simulink model "simulink_jacoviano"  (R2018b)
settings: Solver=VariableStepAuto  StartTime=0.0  StopTime=10.0  RelTol=1e-3
settings Model: Creator=aland  LastModifiedBy=aland

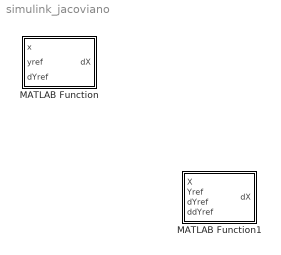
== system simulink_jacoviano ==
  MATLAB Function : MATLAB Function  TreatAsAtomicUnit=on
  MATLAB Function1 : MATLAB Function  TreatAsAtomicUnit=on

== matlab function simulink_jacoviano/MATLAB Function1 ==
  data: X input; dX output; Yref input; dYref input; ddYref input
function dX = simulink_motor(X, Yref, dYref, ddYref)

%MATRICES DEL MOTOR
Ra = 11.24;
La = 2.713e-3;
Kb = 14.87e-3;
Kt = Kb;
bm = 2.01e-6;
Jm = 2779.56e-9;

A = [-Ra/La -Kb/La;Kt/Jm -bm/Jm];
B = [1/La;0];
C = [0 1];

x1 = X(1); x2 = X(2);

e2 = Yref - x2;
de2 = dYref - (Kt/Jm)*x1 + (bm/Jm)*x2;

X1ref = (Jm/Kt)*(dYref + (bm/Jm)*x2 - k2*e2);
dX1ref = (Jm/Kt)*(-k2*de2 + ddYref +  (bm/Jm)*A(2,:)*X);

e1 = X1ref - x1;
U = (La)*(dX1ref + (Ra/La)*x1 + (Kb/La)*x2 - k1*e1);
dX = A*X + B*U;

== matlab function simulink_jacoviano/MATLAB Function ==
  data: x input; dX output; yref input; dYref input
function dX = simulink_jacobiano(x, yref,dYref)

%Parametros del sistema
d = [0.2703 0 0.3644 0 0.3743 0 0.2295]; %metros
a = [0.069 0 0.069 0 0.01 0 0]; %matros
alpha = [-pi/2 pi/2 -pi/2 pi/2 -pi/2 pi/2 0]; %radianes

T = D_H(x0(1:7),a,alpha,d,0,7);
J = jacobiano(T);
Jv = J(4:6,:);

e = yref - x(8:10);
U = pinv(Jv)*(dYref - Ke*e);
    
%ODE's
dX = [U;Jv*U];
